simulink model "PID"  (R2020a)
settings: Solver=VariableStepAuto  StartTime=0.0  StopTime=1  RelTol=1e-3
model workspace (MAT data in the model file):
  Kd = Simulink.Parameter
  Kd.Value = 0.000895
  Kd.DataType = 'auto'
  Kd.Dimensions = [1 1]
  Ki = Simulink.Parameter
  Ki.Value = 0.39
  Ki.DataType = 'auto'
  Ki.Dimensions = [1 1]
  Kp = Simulink.Parameter
  Kp.Value = 0.0121
  Kp.DataType = 'auto'
  Kp.Dimensions = [1 1]
  Ts = Simulink.Parameter
  Ts.Value = 0.01
  Ts.DataType = 'auto'
  Ts.Dimensions = [1 1]
undefined symbols (not defined in the file): DiscIntNeverNeededParam
libraries: simulink x1
settings Model: Creator=Lenovo  LastModifiedBy=Lenovo

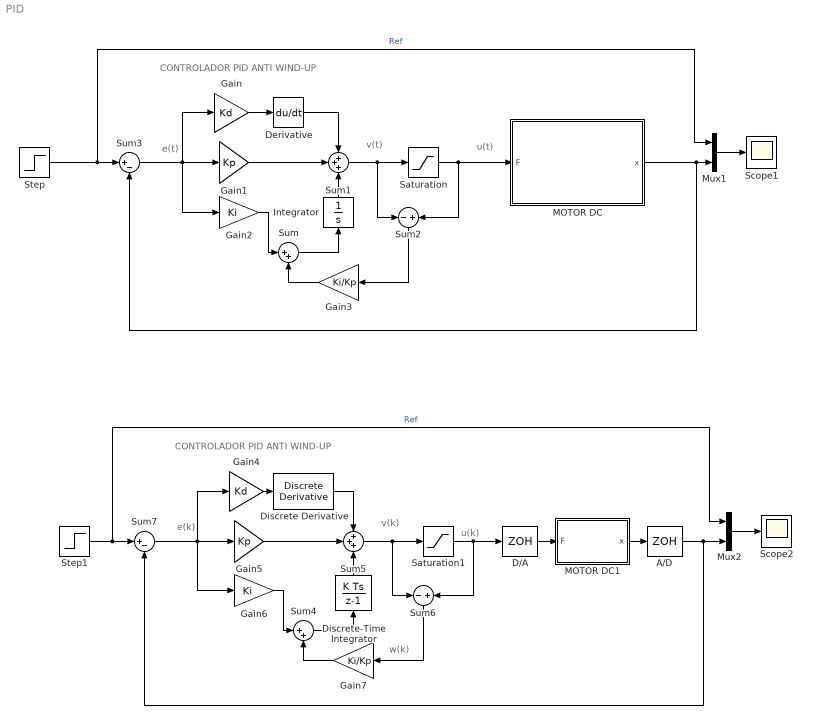
== system PID ==
  note: v(t)
  note: CONTROLADOR PID ANTI WIND-UP
  note: e(t)
  note: u(t)
  note: u(k)
  note: CONTROLADOR PID ANTI WIND-UP
  note: e(k)
  note: v(k)
  note: w(k)
  A/D : ZeroOrderHold  SampleTime=Ts
  D/A : ZeroOrderHold  SampleTime=Ts
  Derivative : Derivative
  Discrete Derivative : simulink/Discrete/Discrete Derivative  gainval=1.0  ICPrevScaledInput=0.0  OutMin=[]  OutMax=[]  OutDataType=fixdt(1, 16)  OutScaling=2^-10  DoSatur=off
  Discrete-Time Integrator : DiscreteIntegrator  SampleTime=Ts  ICPrevOutput=DiscIntNeverNeededParam  ICPrevScaledInput=DiscIntNeverNeededParam
  Gain : Gain  Gain=Kd
  Gain1 : Gain  Gain=Kp
  Gain2 : Gain  Gain=Ki
  Gain3 : Gain  Gain=Ki/Kp
  Gain4 : Gain  Gain=Kd
  Gain5 : Gain  Gain=Kp
  Gain6 : Gain  Gain=Ki
  Gain7 : Gain  Gain=Ki/Kp
  Integrator : Integrator
  MOTOR DC : Subsystem
  MOTOR DC1 : Subsystem
  Mux1 : Mux  Inputs=2
  Mux2 : Mux  Inputs=2
  Saturation : Saturate  UpperLimit=1000  LowerLimit=0
  Saturation1 : Saturate  UpperLimit=20  LowerLimit=0
  Scope1 : Scope
  Scope2 : Scope
  Step : Step  Time=0  After=10  SampleTime=0
  Step1 : Step  Time=0  SampleTime=0
  Sum : Sum  Inputs=|++
  Sum1 : Sum  Inputs=+++
  Sum2 : Sum  Inputs=-+
  Sum3 : Sum  Inputs=|+-
  Sum4 : Sum  Inputs=|++
  Sum5 : Sum  Inputs=+++
  Sum6 : Sum  Inputs=-+
  Sum7 : Sum  Inputs=|+-
  wires:
  MOTOR DC/1(x) -> Mux1/2, Sum3/2
  Saturation/1 -> MOTOR DC/1(F), Sum2/2
  Gain1/1 -> Sum1/2
  Sum/1 -> Integrator/1
  Integrator/1 -> Sum1/3
  Gain/1 -> Derivative/1
  Gain2/1 -> Sum/1
  Sum1/1 -> Sum2/1, Saturation/1
  Derivative/1 -> Sum1/1
  Mux1/1 -> Scope1/1
  Step/1 -> Mux1/1, Sum3/1  "Ref"
  Gain3/1 -> Sum/2
  Sum2/1 -> Gain3/1
  Sum3/1 -> Gain2/1, Gain/1, Gain1/1
  Sum7/1 -> Gain6/1, Gain4/1, Gain5/1
  Gain7/1 -> Sum4/2
  Sum5/1 -> Sum6/1, Saturation1/1
  Discrete-Time Integrator/1 -> Sum5/3
  Step1/1 -> Mux2/1, Sum7/1  "Ref"
  Mux2/1 -> Scope2/1
  Discrete Derivative/1 -> Sum5/1
  Sum6/1 -> Gain7/1
  Gain6/1 -> Sum4/1
  Gain4/1 -> Discrete Derivative/1
  Saturation1/1 -> D/A/1, Sum6/2
  Gain5/1 -> Sum5/2
  Sum4/1 -> Discrete-Time Integrator/1
  D/A/1 -> MOTOR DC1/1(F)
  MOTOR DC1/1(x) -> A/D/1
  A/D/1 -> Sum7/2, Mux2/2

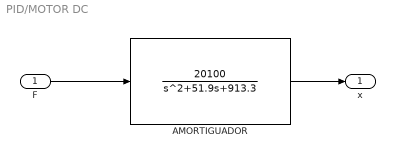
== system PID/MOTOR DC ==
  F : Inport
  AMORTIGUADOR : TransferFcn  Numerator=[20100]  Denominator="[1   51.9  913.3]"
  x : Outport
  wires:
  F/1 -> AMORTIGUADOR/1
  AMORTIGUADOR/1 -> x/1

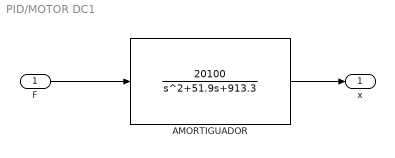
== system PID/MOTOR DC1 ==
  F : Inport
  AMORTIGUADOR : TransferFcn  Numerator=[20100]  Denominator="[1   51.9  913.3]"
  x : Outport
  wires:
  F/1 -> AMORTIGUADOR/1
  AMORTIGUADOR/1 -> x/1
